simulink model "SSB_Modulation"  (R2019b)
settings: Solver=VariableStepAuto  StartTime=0.0  StopTime=0.008  RelTol=1e-3
libraries: dsparch4 x1
settings Model: Creator=Lenovo  LastModifiedBy=Lenovo

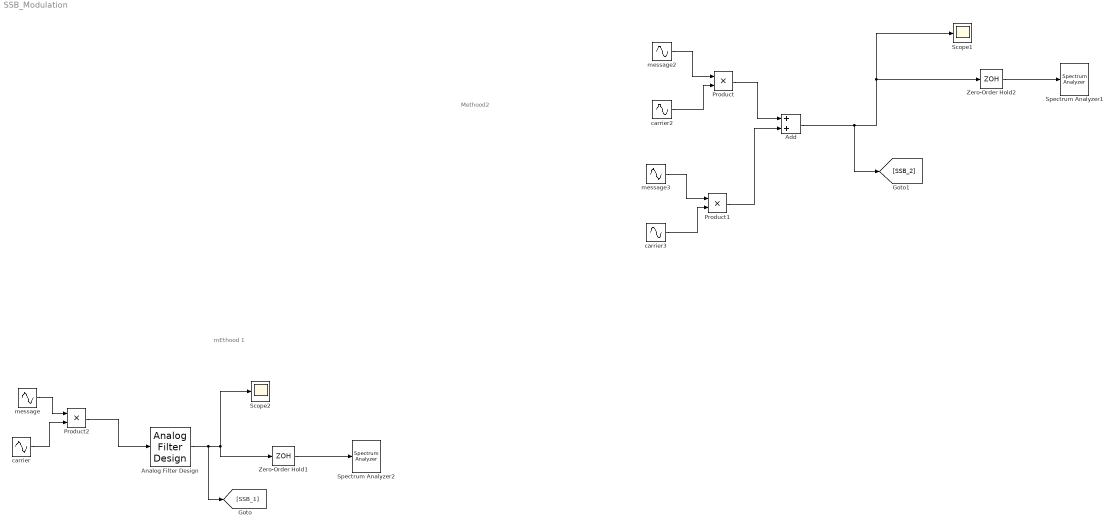
== system SSB_Modulation ==
  note: Methood2
  note: mEthood 1
  Add : Sum
  Analog Filter Design : dsparch4/Analog Filter Design  method=Butterworth  filttype=Bandpass  N=8  Wlo=2*pi*15000  Whi=2*pi*15000+2*pi*1000  Rp=2  Rs=40
  Product : Product
  Product1 : Product
  Product2 : Product
  Scope1 : Scope
  Scope2 : Scope
  Spectrum Analyzer1 : SpectrumAnalyzer
  Spectrum Analyzer2 : SpectrumAnalyzer
  Zero-Order Hold1 : ZeroOrderHold  SampleTime=1/(10*1e3)
  Zero-Order Hold2 : ZeroOrderHold  SampleTime=1/(10*1e3)
  carrier : Sin  Frequency=2*pi*15000  SampleTime=0
  carrier2 : Sin  Frequency=2*pi*15000  SampleTime=0
  carrier3 : Sin  Frequency=2*pi*15000  SampleTime=0
  message : Sin  Amplitude=0.85  Frequency=2*pi*1000  SampleTime=0
  message2 : Sin  Amplitude=0.85  Frequency=2*pi*1000  SampleTime=0
  message3 : Sin  Amplitude=0.85  Frequency=2*pi*1000  SampleTime=0
  wires:
  carrier2/1 -> Product/2
  message2/1 -> Product/1
  Zero-Order Hold2/1 -> Spectrum Analyzer1/1
  carrier3/1 -> Product1/2
  message3/1 -> Product1/1
  Product/1 -> Add/1
  Product1/1 -> Add/2
  Add/1 -> [SSB_2], Zero-Order Hold2/1, Scope1/1
  Zero-Order Hold1/1 -> Spectrum Analyzer2/1
  message/1 -> Product2/1
  carrier/1 -> Product2/2
  Product2/1 -> Analog Filter Design/1
  Analog Filter Design/1 -> [SSB_1], Scope2/1, Zero-Order Hold1/1
